simulink model "Question2"  (R2025b)
settings: Solver=VariableStepAuto  StartTime=0.0  StopTime=10.0  RelTol=1e-3
values from neighbouring files (symbols this model uses):
  g = 9.81    [script_devoir2.m]
  Kdx = -0.367    [script_devoir2.m]
  Kdy = 15000    [script_devoir2.m]
  Kix = -0.176    [script_devoir2.m]
  Kiy = 125000    [script_devoir2.m]
  Kpx = -0.440    (= -0.44)    [script_devoir2.m]
  Kpy = 75000    [script_devoir2.m]
  m = 1000    [script_devoir2.m]
settings Model: Creator=Louis  LastModifiedBy=Louis

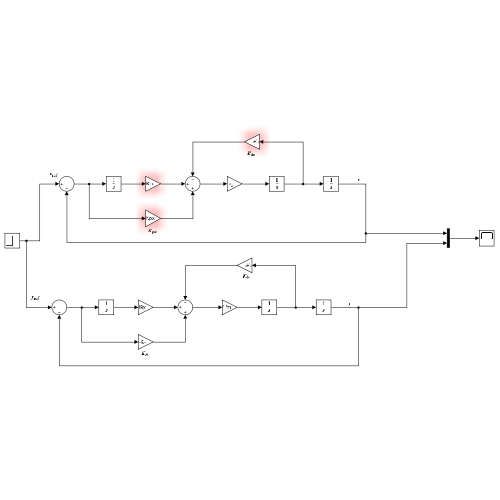
[thumbnail: Simulink's stored preview of the top-level diagram]
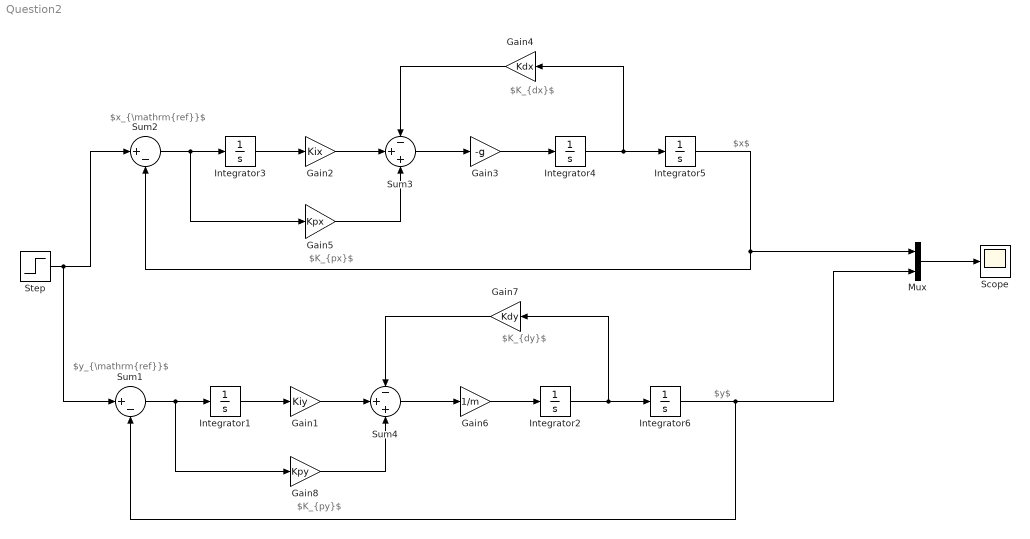
== system Question2 ==
  note: $x$
  note: $K_{py}$
  note: $y$
  note: $K_{px}$
  note: $K_{dy}$
  note: $x_{\mathrm{ref}}$
  note: $y_{\mathrm{ref}}$
  note: $K_{dx}$
  Gain1 : Gain  Gain=Kiy
  Gain2 : Gain  Gain=Kix
  Gain3 : Gain  Gain=-g
  Gain4 : Gain  Gain=Kdx
  Gain5 : Gain  Gain=Kpx
  Gain6 : Gain  Gain=1/m
  Gain7 : Gain  Gain=Kdy
  Gain8 : Gain  Gain=Kpy
  Integrator{1..6} (6 alike) : Integrator
  Mux : Mux  Inputs=2
  Scope : Scope
  Step : Step  Time=0  SampleTime=0
  Sum1 : Sum  Inputs=|+-
  Sum2 : Sum  Inputs=|+-
  Sum3 : Sum  Inputs=-++
  Sum4 : Sum  Inputs=-++
  wires:
  Gain1/1 -> Sum4/2
  Integrator4/1 -> Gain4/1, Integrator5/1
  Integrator2/1 -> Gain7/1, Integrator6/1
  Sum2/1 -> Gain5/1, Integrator3/1
  Gain7/1 -> Sum4/1
  Gain5/1 -> Sum3/3
  Sum3/1 -> Gain3/1
  Gain8/1 -> Sum4/3
  Gain2/1 -> Sum3/2
  Gain3/1 -> Integrator4/1
  Sum1/1 -> Gain8/1, Integrator1/1
  Integrator1/1 -> Gain1/1
  Integrator6/1 -> Mux/2, Sum1/2
  Step/1 -> Sum2/1, Sum1/1
  Integrator3/1 -> Gain2/1
  Integrator5/1 -> Mux/1, Sum2/2
  Gain4/1 -> Sum3/1
  Gain6/1 -> Integrator2/1
  Sum4/1 -> Gain6/1
  Mux/1 -> Scope/1
